simulink model "IEEE_39bus_genout"  (R2021a)
settings: Solver=ode3  StartTime=0.0  StopTime=100  FixedStep=Ts  MaxStep=1/60  RelTol=1e-2  AbsTol=1e-1
PreLoadFcn:
  | Ts=50e-6; ssn_ieee39_params; dec=20;
InitFcn:
  | Ts=50e-6; ssn_ieee39_params; dec=20;
values from neighbouring files (symbols this model uses):
  f = 50    [ssn_ieee39_params_ctrl.m]
  fNom = f    (= 60)    [ssn_ieee39_params_ctrl.m]
  ILR = 5.02    [ssn_ieee39_params_ctrl.m]
  IQMIN = 0.1    [ssn_ieee39_params_ctrl.m]
  ISCLIM = 1    [ssn_ieee39_params_ctrl.m]
  ITFpu = 1.10    (= 1.1)    [ssn_ieee39_params_ctrl.m]
  K = 1    [ssn_ieee39_params_ctrl.m]
  K1 = 1    [ssn_ieee39_params_ctrl.m]
  K2 = 2    [ssn_ieee39_params_ctrl.m]
  KCL = 1.04    [ssn_ieee39_params_ctrl.m]
  KFB = 0    [ssn_ieee39_params_ctrl.m]
  KFF = 1    [ssn_ieee39_params_ctrl.m]
  KFIX = 1    [ssn_ieee39_params_ctrl.m]
  KG = 1    [ssn_ieee39_params_ctrl.m]
  KIA = 59.91    [ssn_ieee39_params_ctrl.m]
  KIOEX = 0.0303    [ssn_ieee39_params_ctrl.m]
  KIUEX = 0.0303    [ssn_ieee39_params_ctrl.m]
  KIUOEX = 1    [ssn_ieee39_params_ctrl.m]
  KIUUEX = 1    [ssn_ieee39_params_ctrl.m]
  KLR = 22.47    [ssn_ieee39_params_ctrl.m]
  KM = 1    [ssn_ieee39_params_ctrl.m]
  KOEL = 0.24    [ssn_ieee39_params_ctrl.m]
  Kp = 1    [ssn_ieee39_params_ctrl.m]
  KPA = 30    [ssn_ieee39_params_ctrl.m]
  KPOEL = 1    [ssn_ieee39_params_ctrl.m]
  KPOEX = 0    [ssn_ieee39_params_ctrl.m]
  KPUEX = 0    [ssn_ieee39_params_ctrl.m]
  KSCALE = 0.319    [ssn_ieee39_params_ctrl.m]
  KUF = 0    [ssn_ieee39_params_ctrl.m]
  KUI = 0.001    [ssn_ieee39_params_ctrl.m]
  KUL = 0.24    [ssn_ieee39_params_ctrl.m]
  s = 10    [ssn_ieee39_params_ctrl.m]
  TA = 0.01    [ssn_ieee39_params_ctrl.m]
  Tadj = 0    [ssn_ieee39_params_ctrl.m]
  taps = [1 1 1.07 1.07 1.009 1.025 1 1.025 1.025 1.025]*1    [ssn_ieee39_params_ctrl.m]
  TF = 0.02    [ssn_ieee39_params_ctrl.m]
  TG = 0.024    [ssn_ieee39_params_ctrl.m]
  TINV = 0    [ssn_ieee39_params_ctrl.m]
  TIT = 0.1    [ssn_ieee39_params_ctrl.m]
  TL_10_11_len = 14    [ssn_ieee39_params_ctrl.m]
  TL_10_13_len = 14    [ssn_ieee39_params_ctrl.m]
  TL_13_14_len = 32    [ssn_ieee39_params_ctrl.m]
  TL_14_15_len = 70    [ssn_ieee39_params_ctrl.m]
  TL_15_16_len = 31.5    [ssn_ieee39_params_ctrl.m]
  TL_16_17_len = 26    [ssn_ieee39_params_ctrl.m]
  TL_16_19_len = 61    [ssn_ieee39_params_ctrl.m]
  TL_16_21_len = 46    [ssn_ieee39_params_ctrl.m]
  TL_16_24_len = 15    [ssn_ieee39_params_ctrl.m]
  TL_17_18_len = 26    [ssn_ieee39_params_ctrl.m]
  TL_17_27_len = 59    [ssn_ieee39_params_ctrl.m]
  TL_1_2_len = 134    [ssn_ieee39_params_ctrl.m]
  TL_1_39_len = 105    [ssn_ieee39_params_ctrl.m]
  TL_21_22_len = 47    [ssn_ieee39_params_ctrl.m]
  TL_22_23_len = 33    [ssn_ieee39_params_ctrl.m]
  TL_24_23_len = 88    [ssn_ieee39_params_ctrl.m]
  TL_25_26_len = 101    [ssn_ieee39_params_ctrl.m]
  TL_26_27_len = 46.5    [ssn_ieee39_params_ctrl.m]
  TL_26_28_len = 151    [ssn_ieee39_params_ctrl.m]
  TL_26_29_len = 200    [ssn_ieee39_params_ctrl.m]
  TL_28_29_len = 48    [ssn_ieee39_params_ctrl.m]
  TL_2_25_len = 28    [ssn_ieee39_params_ctrl.m]
  TL_2_2_len = 49    [ssn_ieee39_params_ctrl.m]
  TL_3_18_len = 42    [ssn_ieee39_params_ctrl.m]
  TL_3_4_len = 53    [ssn_ieee39_params_ctrl.m]
  TL_4_14_len = 33    [ssn_ieee39_params_ctrl.m]
  TL_4_5_len = 32.5    [ssn_ieee39_params_ctrl.m]
  TL_5_6_len = 14    [ssn_ieee39_params_ctrl.m]
  TL_5_8_len = 32    [ssn_ieee39_params_ctrl.m]
  TL_6_11_len = 26.5    [ssn_ieee39_params_ctrl.m]
  TL_6_7_len = 25.5    [ssn_ieee39_params_ctrl.m]
  TL_7_8_len = 15    [ssn_ieee39_params_ctrl.m]
  TL_8_9_len = 93    [ssn_ieee39_params_ctrl.m]
  TL_9_39_len = 136    [ssn_ieee39_params_ctrl.m]
  TOEL = 5.00    (= 5)    [ssn_ieee39_params_ctrl.m]
  TQREF = 0    [ssn_ieee39_params_ctrl.m]
  TQSCL = 0.012    [ssn_ieee39_params_ctrl.m]
  Ts_PMU = 1/1000    (= 0.001)    [ssn_ieee39_params_ctrl.m]
  TU1 = 0    [ssn_ieee39_params_ctrl.m]
  TU2 = 0    [ssn_ieee39_params_ctrl.m]
  TU3 = 0    [ssn_ieee39_params_ctrl.m]
  TU4 = 0    [ssn_ieee39_params_ctrl.m]
  TUL = 0    [ssn_ieee39_params_ctrl.m]
  TUP = 0.050    (= 0.05)    [ssn_ieee39_params_ctrl.m]
  TUQ = .005    (= 0.005)    [ssn_ieee39_params_ctrl.m]
  TUV = 0.2    [ssn_ieee39_params_ctrl.m]
  VAAMAX = VAMAX    (= 7.05)    [ssn_ieee39_params_ctrl.m]
  VAMAX = 7.05    [ssn_ieee39_params_ctrl.m]
  VAMIN = -6.11    [ssn_ieee39_params_ctrl.m]
  VBMAX = 999    [ssn_ieee39_params_ctrl.m]
  VF = 0    [ssn_ieee39_params_ctrl.m]
  VFB = 0    [ssn_ieee39_params_ctrl.m]
  VMMAX = 7.05    [ssn_ieee39_params_ctrl.m]
  VMMIN = -6.11    [ssn_ieee39_params_ctrl.m]
  VOELmax1 = 0.2353    [ssn_ieee39_params_ctrl.m]
  VOELmax2 = 0.0    (= 0)    [ssn_ieee39_params_ctrl.m]
  VOELmin1 = -0.24    [ssn_ieee39_params_ctrl.m]
  VOELmin2 = -1.0    (= -1)    [ssn_ieee39_params_ctrl.m]
  VRMAX = 7.05    [ssn_ieee39_params_ctrl.m]
  VRMIN = -6.11    [ssn_ieee39_params_ctrl.m]
  VSCLmax = 0.20    (= 0.2)    [ssn_ieee39_params_ctrl.m]
  VSCLmin = -0.10    (= -0.1)    [ssn_ieee39_params_ctrl.m]
  VUELmax1 = 1    [ssn_ieee39_params_ctrl.m]
  VUELmax2 = 1    [ssn_ieee39_params_ctrl.m]
  VUELmin1 = -1    [ssn_ieee39_params_ctrl.m]
  VUELmin2 = -1    [ssn_ieee39_params_ctrl.m]
  VUImax = 1    [ssn_ieee39_params_ctrl.m]
  VUImin = -1    [ssn_ieee39_params_ctrl.m]
undefined symbols (not defined in the file or in its folder): D1, Delta, MOV_segment9, powergui
libraries: spsThreePhaseVIMeasurementLib x42, slpidlib x40, powerlib_extras x30, op_dpl_lib x30, simulink_extras x20, spsST2AModel x20, spsThreePhaseParallelRLCLoadLib x19, spsThreePhaseTransformerTwoWindingsLib x13, spsSynchronousMachinepuStandardLib x10, simulink x10, spsPower3phInstantaneousLib x10, spsThreePhasePISectionLineLib x7
(part 4 of 12)

== system IEEE_39bus_genout/SM_master/PMU_Vpos_60Hz7 ==
  abc : Inport  PortDimensions=3
  1 / sqrt of 2 : Gain  Gain=1/sqrt(2)  OutDataTypeStr=Inherit: Same as input  ParamDataTypeStr=Inherit: Same as input
  Cartesian to Polar : simulink_extras/Transformations/Cartesian to Polar
  Demux : Demux  Outputs=3
      settings: DisplayOption=none
  Discrete Mean value1 : powerlib_extras/Discrete Measurements/Discrete  Mean value  Freq=Freq  Vinit=Real_Init  Ts=Ts
      settings: SourceProductBaseCode=PS
  Discrete Mean value2 : powerlib_extras/Discrete Measurements/Discrete  Mean value  Freq=Freq  Vinit=Imag_Init  Ts=Ts
      settings: SourceProductBaseCode=PS
  Discrete Derivative : simulink/Discrete/Discrete Derivative  gainval=1.0  ICPrevScaledInput=0.0  OutMin=[]  OutMax=[]  OutDataType=fixdt(1, 16)  OutScaling=2^-10  DoSatur=off
  Gain : Gain  Gain=2*pi*Freq  SaturateOnIntegerOverflow=on  OutDataTypeStr=Inherit: Same as input  ParamDataTypeStr=Inherit: Same as input
  Mux : Mux  Inputs=2
  Rad->Deg. : Gain  Gain=180/pi  SaturateOnIntegerOverflow=on  OutDataTypeStr=Inherit: Same as input  ParamDataTypeStr=Inherit: Same as input
  Sum : Sum  Inputs=|++  OutDataTypeStr=Inherit: Same as first input
  Terminator : Terminator
  Trigonometric Function : Trigonometry
  Trigonometric Function1 : Trigonometry  Operator=cos
  abc_to_dq0 Transformation : powerlib_extras/Measurements/abc_to_dq0 Transformation
      settings: SourceProductBaseCode=PS
  fo : Constant  Value=2*pi*Freq
  t : DigitalClock  SampleTime=Ts
  Mag : Outport
  Phase : Outport  Port=2
  freq : Outport  Port=3
  dfdt : Outport  Port=4
  wires:
  Cartesian to Polar/2 -> Rad->Deg./1, Discrete Derivative/1
  Gain/1 -> Trigonometric Function1/1, Trigonometric Function/1
  t/1 -> Gain/1
  abc/1 -> abc_to_dq0 Transformation/1
  Mux/1 -> abc_to_dq0 Transformation/2
  Discrete Mean value1/1 -> Cartesian to Polar/1  "Real"
  Rad->Deg./1 -> Phase/1
  Discrete Mean value2/1 -> Cartesian to Polar/2  "Real"
  abc_to_dq0 Transformation/1 -> Demux/1
  Demux/3 -> Terminator/1
  Demux/2 -> Discrete Mean value2/1
  Demux/1 -> Discrete Mean value1/1
  Trigonometric Function/1 -> Mux/1
  Trigonometric Function1/1 -> Mux/2
  Cartesian to Polar/1 -> 1 / sqrt of 2/1
  1 / sqrt of 2/1 -> Mag/1
  Discrete Derivative/1 -> Sum/2, dfdt/1
  fo/1 -> Sum/1
  Sum/1 -> freq/1

== system IEEE_39bus_genout/SM_master/PMU_Vpos_60Hz8 ==
  abc : Inport  PortDimensions=3
  1 / sqrt of 2 : Gain  Gain=1/sqrt(2)  OutDataTypeStr=Inherit: Same as input  ParamDataTypeStr=Inherit: Same as input
  Cartesian to Polar : simulink_extras/Transformations/Cartesian to Polar
  Demux : Demux  Outputs=3
      settings: DisplayOption=none
  Discrete Mean value1 : powerlib_extras/Discrete Measurements/Discrete  Mean value  Freq=Freq  Vinit=Real_Init  Ts=Ts
      settings: SourceProductBaseCode=PS
  Discrete Mean value2 : powerlib_extras/Discrete Measurements/Discrete  Mean value  Freq=Freq  Vinit=Imag_Init  Ts=Ts
      settings: SourceProductBaseCode=PS
  Discrete Derivative : simulink/Discrete/Discrete Derivative  gainval=1.0  ICPrevScaledInput=0.0  OutMin=[]  OutMax=[]  OutDataType=fixdt(1, 16)  OutScaling=2^-10  DoSatur=off
  Gain : Gain  Gain=2*pi*Freq  SaturateOnIntegerOverflow=on  OutDataTypeStr=Inherit: Same as input  ParamDataTypeStr=Inherit: Same as input
  Mux : Mux  Inputs=2
  Rad->Deg. : Gain  Gain=180/pi  SaturateOnIntegerOverflow=on  OutDataTypeStr=Inherit: Same as input  ParamDataTypeStr=Inherit: Same as input
  Sum : Sum  Inputs=|++  OutDataTypeStr=Inherit: Same as first input
  Terminator : Terminator
  Trigonometric Function : Trigonometry
  Trigonometric Function1 : Trigonometry  Operator=cos
  abc_to_dq0 Transformation : powerlib_extras/Measurements/abc_to_dq0 Transformation
      settings: SourceProductBaseCode=PS
  fo : Constant  Value=2*pi*Freq
  t : DigitalClock  SampleTime=Ts
  Mag : Outport
  Phase : Outport  Port=2
  freq : Outport  Port=3
  dfdt : Outport  Port=4
  wires:
  Cartesian to Polar/2 -> Rad->Deg./1, Discrete Derivative/1
  Gain/1 -> Trigonometric Function1/1, Trigonometric Function/1
  t/1 -> Gain/1
  abc/1 -> abc_to_dq0 Transformation/1
  Mux/1 -> abc_to_dq0 Transformation/2
  Discrete Mean value1/1 -> Cartesian to Polar/1  "Real"
  Rad->Deg./1 -> Phase/1
  Discrete Mean value2/1 -> Cartesian to Polar/2  "Real"
  abc_to_dq0 Transformation/1 -> Demux/1
  Demux/3 -> Terminator/1
  Demux/2 -> Discrete Mean value2/1
  Demux/1 -> Discrete Mean value1/1
  Trigonometric Function/1 -> Mux/1
  Trigonometric Function1/1 -> Mux/2
  Cartesian to Polar/1 -> 1 / sqrt of 2/1
  1 / sqrt of 2/1 -> Mag/1
  Discrete Derivative/1 -> Sum/2, dfdt/1
  fo/1 -> Sum/1
  Sum/1 -> freq/1

== system IEEE_39bus_genout/SM_master/PMU_Vpos_60Hz9 ==
  abc : Inport  PortDimensions=3
  1 / sqrt of 2 : Gain  Gain=1/sqrt(2)  OutDataTypeStr=Inherit: Same as input  ParamDataTypeStr=Inherit: Same as input
  Cartesian to Polar : simulink_extras/Transformations/Cartesian to Polar
  Demux : Demux  Outputs=3
      settings: DisplayOption=none
  Discrete Mean value1 : powerlib_extras/Discrete Measurements/Discrete  Mean value  Freq=Freq  Vinit=Real_Init  Ts=Ts
      settings: SourceProductBaseCode=PS
  Discrete Mean value2 : powerlib_extras/Discrete Measurements/Discrete  Mean value  Freq=Freq  Vinit=Imag_Init  Ts=Ts
      settings: SourceProductBaseCode=PS
  Discrete Derivative : simulink/Discrete/Discrete Derivative  gainval=1.0  ICPrevScaledInput=0.0  OutMin=[]  OutMax=[]  OutDataType=fixdt(1, 16)  OutScaling=2^-10  DoSatur=off
  Gain : Gain  Gain=2*pi*Freq  SaturateOnIntegerOverflow=on  OutDataTypeStr=Inherit: Same as input  ParamDataTypeStr=Inherit: Same as input
  Mux : Mux  Inputs=2
  Rad->Deg. : Gain  Gain=180/pi  SaturateOnIntegerOverflow=on  OutDataTypeStr=Inherit: Same as input  ParamDataTypeStr=Inherit: Same as input
  Sum : Sum  Inputs=|++  OutDataTypeStr=Inherit: Same as first input
  Terminator : Terminator
  Trigonometric Function : Trigonometry
  Trigonometric Function1 : Trigonometry  Operator=cos
  abc_to_dq0 Transformation : powerlib_extras/Measurements/abc_to_dq0 Transformation
      settings: SourceProductBaseCode=PS
  fo : Constant  Value=2*pi*Freq
  t : DigitalClock  SampleTime=Ts
  Mag : Outport
  Phase : Outport  Port=2
  freq : Outport  Port=3
  dfdt : Outport  Port=4
  wires:
  Cartesian to Polar/2 -> Rad->Deg./1, Discrete Derivative/1
  Gain/1 -> Trigonometric Function1/1, Trigonometric Function/1
  t/1 -> Gain/1
  abc/1 -> abc_to_dq0 Transformation/1
  Mux/1 -> abc_to_dq0 Transformation/2
  Discrete Mean value1/1 -> Cartesian to Polar/1  "Real"
  Rad->Deg./1 -> Phase/1
  Discrete Mean value2/1 -> Cartesian to Polar/2  "Real"
  abc_to_dq0 Transformation/1 -> Demux/1
  Demux/3 -> Terminator/1
  Demux/2 -> Discrete Mean value2/1
  Demux/1 -> Discrete Mean value1/1
  Trigonometric Function/1 -> Mux/1
  Trigonometric Function1/1 -> Mux/2
  Cartesian to Polar/1 -> 1 / sqrt of 2/1
  1 / sqrt of 2/1 -> Mag/1
  Discrete Derivative/1 -> Sum/2, dfdt/1
  fo/1 -> Sum/1
  Sum/1 -> freq/1

== system IEEE_39bus_genout/SM_master/Power ==
  Mux : Mux  Inputs=10
  Power (3ph, Instantaneous){1..10} (10 alike) : spsPower3phInstantaneousLib/Power (3ph, Instantaneous)
  Scope{1..10} (10 alike) : Scope  NumInputPorts=2
  to PU{1..20} (20 alike) : Gain
  Pgen : Outport
  tag scope: PG_10=global, PG_1=global, PG_2=global, PG_3=global, PG_4=global, PG_5=global, PG_6=global, PG_7=global, PG_8=global, PG_9=global
  wires:
  [Iabc_30] -> "Power (3ph, Instantaneous)1"/2
  to PU2/1 -> Scope7/2, [QG_10]
  [Vabc_30] -> "Power (3ph, Instantaneous)1"/1
  "Power (3ph, Instantaneous)4"/2 -> to PU9/1
  to PU8/1 -> [PG_8], Scope4/1
  "Power (3ph, Instantaneous)1"/1 -> to PU1/1
  "Power (3ph, Instantaneous)1"/2 -> to PU2/1
  "Power (3ph, Instantaneous)4"/1 -> to PU8/1
  [Vabc_37] -> "Power (3ph, Instantaneous)4"/1
  to PU1/1 -> Scope7/1, [PG_10]
  [Iabc_37] -> "Power (3ph, Instantaneous)4"/2
  to PU9/1 -> [QG_8], Scope4/2
  to PU6/1 -> Scope1/2, [QG_9]
  [Iabc_29] -> "Power (3ph, Instantaneous)3"/2
  to PU3/1 -> [PG_1], Scope2/1
  [Vabc_29] -> "Power (3ph, Instantaneous)3"/1
  "Power (3ph, Instantaneous)3"/1 -> to PU5/1
  "Power (3ph, Instantaneous)2"/2 -> to PU4/1
  "Power (3ph, Instantaneous)2"/1 -> to PU3/1
  to PU5/1 -> Scope1/1, [PG_9]
  "Power (3ph, Instantaneous)3"/2 -> to PU6/1
  [Vabc_391] -> "Power (3ph, Instantaneous)2"/1
  to PU4/1 -> [QG_1], Scope2/2
  [Iabc_391] -> "Power (3ph, Instantaneous)2"/2
  [Iabc_34] -> "Power (3ph, Instantaneous)6"/2
  to PU12/1 -> Scope5/2, [QG_5]
  [Vabc_34] -> "Power (3ph, Instantaneous)6"/1
  "Power (3ph, Instantaneous)7"/2 -> to PU14/1
  to PU13/1 -> [PG_4], Scope3/1
  "Power (3ph, Instantaneous)6"/1 -> to PU11/1
  "Power (3ph, Instantaneous)6"/2 -> to PU12/1
  "Power (3ph, Instantaneous)7"/1 -> to PU13/1
  [Vabc_33] -> "Power (3ph, Instantaneous)7"/1
  to PU11/1 -> Scope5/1, [PG_5]
  [Iabc_33] -> "Power (3ph, Instantaneous)7"/2
  to PU14/1 -> [QG_4], Scope3/2
  to PU16/1 -> Scope6/2, [QG_2]
  [Iabc_31] -> "Power (3ph, Instantaneous)8"/2
  to PU7/1 -> [PG_3], Scope8/1
  [Vabc_31] -> "Power (3ph, Instantaneous)8"/1
  "Power (3ph, Instantaneous)8"/1 -> to PU15/1
  "Power (3ph, Instantaneous)5"/2 -> to PU10/1
  "Power (3ph, Instantaneous)5"/1 -> to PU7/1
  to PU15/1 -> Scope6/1, [PG_2]
  "Power (3ph, Instantaneous)8"/2 -> to PU16/1
  [Vabc_32] -> "Power (3ph, Instantaneous)5"/1
  to PU10/1 -> [QG_3], Scope8/2
  [Iabc_32] -> "Power (3ph, Instantaneous)5"/2
  [Iabc_35] -> "Power (3ph, Instantaneous)9"/2
  to PU17/1 -> Scope10/2, [QG_6]
  [Vabc_35] -> "Power (3ph, Instantaneous)9"/1
  "Power (3ph, Instantaneous)9"/1 -> to PU20/1
  "Power (3ph, Instantaneous)9"/2 -> to PU17/1
  to PU20/1 -> Scope10/1, [PG_6]
  to PU18/1 -> [PG_7], Scope9/1
  "Power (3ph, Instantaneous)10"/2 -> to PU19/1
  "Power (3ph, Instantaneous)10"/1 -> to PU18/1
  [Vabc_36] -> "Power (3ph, Instantaneous)10"/1
  to PU19/1 -> [QG_7], Scope9/2
  [Iabc_36] -> "Power (3ph, Instantaneous)10"/2
  [PG_1] -> Mux/1
  [PG_2] -> Mux/2
  [PG_3] -> Mux/3
  [PG_4] -> Mux/4
  [PG_5] -> Mux/5
  [PG_6] -> Mux/6
  [PG_7] -> Mux/7
  [PG_8] -> Mux/8
  [PG_9] -> Mux/9
  [PG_10] -> Mux/10
  Mux/1 -> Pgen/1

== system IEEE_39bus_genout/SM_master/Snubber circuit ==
  Snubber 2 : spsThreePhaseSeriesRLCLoadLib/Three-Phase Series RLC Load  LConnTagsString=A|B|C  Configuration=Y (grounded)  NominalVoltage=20000  Vabc=[1e3 1e3 1e3]  Vabcp=[1e3 1e3 1e3]  NominalFrequency=60  UnbalancedPower=off  ActivePower=1e6  InductivePower=0  CapacitivePower=1e7  Pabc=[10e3 9e3 11e3]  QLabc=[100 90 110]  QCabc=[100 90 110]  Pabcp=[10e3 9e3 11e3]  QLabcp=[100 90 110]  QCabcp=[100 90 110]  Measurements=None  LoadType=constant Z
  Three-Phase Series RLC Branch : spsThreePhaseSeriesRLCBranchLib/Three-Phase Series RLC Branch  LConnTagsString=A|B|C  RConnTagsString=A|B|C  BranchType=R  Resistance=1e10  Inductance=1e-3  Capacitance=1e-6  Measurements=None
  a : PMIOPort  Side=Left
  b : PMIOPort  Port=2  Side=Left
  c : PMIOPort  Port=3  Side=Left
  Conn4 : PMIOPort  Port=4  Side=Right
  connections:
  Snubber 2/LConn3 -- c/RConn1 -- Three-Phase Series RLC Branch/LConn3
  Three-Phase Series RLC Branch/RConn2 -- Conn4/RConn1 -- Three-Phase Series RLC Branch/RConn3 -- Three-Phase Series RLC Branch/RConn1
  Three-Phase Series RLC Branch/LConn2 -- b/RConn1 -- Snubber 2/LConn2
  Three-Phase Series RLC Branch/LConn1 -- a/RConn1 -- Snubber 2/LConn1

== system IEEE_39bus_genout/powergui/EquivalentModel1 ==
  Sources : Subsystem
  State-Space : S-Function  FunctionName=ssn_sfun_v1  Parameters=1,0  SFunctionDeploymentMode=off  EnableBusSupport=off  SFcnStateName=MOV_segment9,MOV_segment9,MOV_segment9,MOV_segment9,MOV_segment9,MOV_segment9,MOV_segment9,MOV_segment9,MOV_segment9,MOV_segment9
      settings: SFcnIsStateOwnerBlock=on
  Yout : Subsystem
  wires:
  State-Space/1 -> Yout/1(v,i)
  Sources/1(u) -> State-Space/1

== system IEEE_39bus_genout/powergui/EquivalentModel10 ==
  Sources : Subsystem
  State-Space : S-Function  FunctionName=ssn_sfun_v1  Parameters=10,0  SFunctionDeploymentMode=off  EnableBusSupport=off  SFcnStateName=MOV_segment9,MOV_segment9,MOV_segment9,MOV_segment9,MOV_segment9,MOV_segment9,MOV_segment9,MOV_segment9,MOV_segment9,MOV_segment9
      settings: SFcnIsStateOwnerBlock=on
  Yout : Subsystem
  wires:
  State-Space/1 -> Yout/1(v,i)
  Sources/1(u) -> State-Space/1

== system IEEE_39bus_genout/powergui/EquivalentModel11 ==
  Sources : Subsystem
  State-Space : S-Function  FunctionName=ssn_sfun_v1  Parameters=11,0  SFunctionDeploymentMode=off  EnableBusSupport=off  SFcnStateName=MOV_segment9,MOV_segment9,MOV_segment9,MOV_segment9,MOV_segment9,MOV_segment9,MOV_segment9,MOV_segment9,MOV_segment9,MOV_segment9
      settings: SFcnIsStateOwnerBlock=on
  Yout : Subsystem
  wires:
  State-Space/1 -> Yout/1(v,i)
  Sources/1(u) -> State-Space/1

== system IEEE_39bus_genout/powergui/EquivalentModel12 ==
  Sources : Subsystem
  State-Space : S-Function  FunctionName=ssn_sfun_v1  Parameters=12,0  SFunctionDeploymentMode=off  EnableBusSupport=off  SFcnStateName=MOV_segment9,MOV_segment9,MOV_segment9,MOV_segment9,MOV_segment9,MOV_segment9,MOV_segment9,MOV_segment9,MOV_segment9,MOV_segment9
      settings: SFcnIsStateOwnerBlock=on
  Yout : Subsystem
  wires:
  State-Space/1 -> Yout/1(v,i)
  Sources/1(u) -> State-Space/1

== system IEEE_39bus_genout/powergui/EquivalentModel13 ==
  Sources : Subsystem
  State-Space : S-Function  FunctionName=ssn_sfun_v1  Parameters=13,0  SFunctionDeploymentMode=off  EnableBusSupport=off  SFcnStateName=MOV_segment9,MOV_segment9,MOV_segment9,MOV_segment9,MOV_segment9,MOV_segment9,MOV_segment9,MOV_segment9,MOV_segment9,MOV_segment9
      settings: SFcnIsStateOwnerBlock=on
  Yout : Subsystem
  wires:
  State-Space/1 -> Yout/1(v,i)
  Sources/1(u) -> State-Space/1

== system IEEE_39bus_genout/powergui/EquivalentModel14 ==
  Sources : Subsystem
  State-Space : S-Function  FunctionName=ssn_sfun_v1  Parameters=14,0  SFunctionDeploymentMode=off  EnableBusSupport=off  SFcnStateName=MOV_segment9,MOV_segment9,MOV_segment9,MOV_segment9,MOV_segment9,MOV_segment9,MOV_segment9,MOV_segment9,MOV_segment9,MOV_segment9
      settings: SFcnIsStateOwnerBlock=on
  Yout : Subsystem
  wires:
  State-Space/1 -> Yout/1(v,i)
  Sources/1(u) -> State-Space/1

== system IEEE_39bus_genout/powergui/EquivalentModel15 ==
  Sources : Subsystem
  State-Space : S-Function  FunctionName=ssn_sfun_v1  Parameters=15,0  SFunctionDeploymentMode=off  EnableBusSupport=off  SFcnStateName=MOV_segment9,MOV_segment9,MOV_segment9,MOV_segment9,MOV_segment9,MOV_segment9,MOV_segment9,MOV_segment9,MOV_segment9,MOV_segment9
      settings: SFcnIsStateOwnerBlock=on
  Yout : Subsystem
  wires:
  State-Space/1 -> Yout/1(v,i)
  Sources/1(u) -> State-Space/1

== system IEEE_39bus_genout/powergui/EquivalentModel16 ==
  Sources : Subsystem
  State-Space : S-Function  FunctionName=ssn_sfun_v1  Parameters=16,0  SFunctionDeploymentMode=off  EnableBusSupport=off  SFcnStateName=MOV_segment9,MOV_segment9,MOV_segment9,MOV_segment9,MOV_segment9,MOV_segment9,MOV_segment9,MOV_segment9,MOV_segment9,MOV_segment9
      settings: SFcnIsStateOwnerBlock=on
  Yout : Subsystem
  wires:
  State-Space/1 -> Yout/1(v,i)
  Sources/1(u) -> State-Space/1

== system IEEE_39bus_genout/powergui/EquivalentModel17 ==
  Sources : Subsystem
  State-Space : S-Function  FunctionName=ssn_sfun_v1  Parameters=17,0  SFunctionDeploymentMode=off  EnableBusSupport=off  SFcnStateName=MOV_segment9,MOV_segment9,MOV_segment9,MOV_segment9,MOV_segment9,MOV_segment9,MOV_segment9,MOV_segment9,MOV_segment9,MOV_segment9
      settings: SFcnIsStateOwnerBlock=on
  Yout : Subsystem
  wires:
  State-Space/1 -> Yout/1(v,i)
  Sources/1(u) -> State-Space/1

== system IEEE_39bus_genout/powergui/EquivalentModel18 ==
  Sources : Subsystem
  State-Space : S-Function  FunctionName=ssn_sfun_v1  Parameters=18,0  SFunctionDeploymentMode=off  EnableBusSupport=off  SFcnStateName=MOV_segment9,MOV_segment9,MOV_segment9,MOV_segment9,MOV_segment9,MOV_segment9,MOV_segment9,MOV_segment9,MOV_segment9,MOV_segment9
      settings: SFcnIsStateOwnerBlock=on
  Yout : Subsystem
  wires:
  State-Space/1 -> Yout/1(v,i)
  Sources/1(u) -> State-Space/1

== system IEEE_39bus_genout/powergui/EquivalentModel19 ==
  Gates : Subsystem
  Sources : Subsystem
  State-Space : S-Function  FunctionName=ssn_sfun_v1  Parameters=19,0  SFunctionDeploymentMode=off  EnableBusSupport=off  SFcnStateName=MOV_segment9,MOV_segment9,MOV_segment9,MOV_segment9,MOV_segment9,MOV_segment9,MOV_segment9,MOV_segment9,MOV_segment9,MOV_segment9
      settings: SFcnIsStateOwnerBlock=on
  Status : Subsystem
  Yout : Subsystem
  wires:
  Gates/1(gates) -> State-Space/2
  Sources/1(u) -> State-Space/1
  State-Space/2 -> Status/1(status)
  State-Space/1 -> Yout/1(v,i)

== system IEEE_39bus_genout/powergui/EquivalentModel2 ==
  Sources : Subsystem
  State-Space : S-Function  FunctionName=ssn_sfun_v1  Parameters=2,0  SFunctionDeploymentMode=off  EnableBusSupport=off  SFcnStateName=MOV_segment9,MOV_segment9,MOV_segment9,MOV_segment9,MOV_segment9,MOV_segment9,MOV_segment9,MOV_segment9,MOV_segment9,MOV_segment9
      settings: SFcnIsStateOwnerBlock=on
  Yout : Subsystem
  wires:
  State-Space/1 -> Yout/1(v,i)
  Sources/1(u) -> State-Space/1

== system IEEE_39bus_genout/powergui/EquivalentModel20 ==
  Sources : Subsystem
  State-Space : S-Function  FunctionName=ssn_sfun_v1  Parameters=20,0  SFunctionDeploymentMode=off  EnableBusSupport=off  SFcnStateName=MOV_segment9,MOV_segment9,MOV_segment9,MOV_segment9,MOV_segment9,MOV_segment9,MOV_segment9,MOV_segment9,MOV_segment9,MOV_segment9
      settings: SFcnIsStateOwnerBlock=on
  Yout : Subsystem
  wires:
  State-Space/1 -> Yout/1(v,i)
  Sources/1(u) -> State-Space/1

== system IEEE_39bus_genout/powergui/EquivalentModel21 ==
  Sources : Subsystem
  State-Space : S-Function  FunctionName=ssn_sfun_v1  Parameters=21,0  SFunctionDeploymentMode=off  EnableBusSupport=off  SFcnStateName=MOV_segment9,MOV_segment9,MOV_segment9,MOV_segment9,MOV_segment9,MOV_segment9,MOV_segment9,MOV_segment9,MOV_segment9,MOV_segment9
      settings: SFcnIsStateOwnerBlock=on
  Yout : Subsystem
  wires:
  State-Space/1 -> Yout/1(v,i)
  Sources/1(u) -> State-Space/1

== system IEEE_39bus_genout/powergui/EquivalentModel22 ==
  Sources : Subsystem
  State-Space : S-Function  FunctionName=ssn_sfun_v1  Parameters=22,0  SFunctionDeploymentMode=off  EnableBusSupport=off  SFcnStateName=MOV_segment9,MOV_segment9,MOV_segment9,MOV_segment9,MOV_segment9,MOV_segment9,MOV_segment9,MOV_segment9,MOV_segment9,MOV_segment9
      settings: SFcnIsStateOwnerBlock=on
  Yout : Subsystem
  wires:
  State-Space/1 -> Yout/1(v,i)
  Sources/1(u) -> State-Space/1

== system IEEE_39bus_genout/powergui/EquivalentModel23 ==
  Sources : Subsystem
  State-Space : S-Function  FunctionName=ssn_sfun_v1  Parameters=23,0  SFunctionDeploymentMode=off  EnableBusSupport=off  SFcnStateName=MOV_segment9,MOV_segment9,MOV_segment9,MOV_segment9,MOV_segment9,MOV_segment9,MOV_segment9,MOV_segment9,MOV_segment9,MOV_segment9
      settings: SFcnIsStateOwnerBlock=on
  Yout : Subsystem
  wires:
  State-Space/1 -> Yout/1(v,i)
  Sources/1(u) -> State-Space/1

== system IEEE_39bus_genout/powergui/EquivalentModel24 ==
  Sources : Subsystem
  State-Space : S-Function  FunctionName=ssn_sfun_v1  Parameters=24,0  SFunctionDeploymentMode=off  EnableBusSupport=off  SFcnStateName=MOV_segment9,MOV_segment9,MOV_segment9,MOV_segment9,MOV_segment9,MOV_segment9,MOV_segment9,MOV_segment9,MOV_segment9,MOV_segment9
      settings: SFcnIsStateOwnerBlock=on
  Yout : Subsystem
  wires:
  State-Space/1 -> Yout/1(v,i)
  Sources/1(u) -> State-Space/1

== system IEEE_39bus_genout/powergui/EquivalentModel3 ==
  Sources : Subsystem
  State-Space : S-Function  FunctionName=ssn_sfun_v1  Parameters=3,0  SFunctionDeploymentMode=off  EnableBusSupport=off  SFcnStateName=MOV_segment9,MOV_segment9,MOV_segment9,MOV_segment9,MOV_segment9,MOV_segment9,MOV_segment9,MOV_segment9,MOV_segment9,MOV_segment9
      settings: SFcnIsStateOwnerBlock=on
  Yout : Subsystem
  wires:
  State-Space/1 -> Yout/1(v,i)
  Sources/1(u) -> State-Space/1

== system IEEE_39bus_genout/powergui/EquivalentModel4 ==
  Sources : Subsystem
  State-Space : S-Function  FunctionName=ssn_sfun_v1  Parameters=4,0  SFunctionDeploymentMode=off  EnableBusSupport=off  SFcnStateName=MOV_segment9,MOV_segment9,MOV_segment9,MOV_segment9,MOV_segment9,MOV_segment9,MOV_segment9,MOV_segment9,MOV_segment9,MOV_segment9
      settings: SFcnIsStateOwnerBlock=on
  Yout : Subsystem
  wires:
  State-Space/1 -> Yout/1(v,i)
  Sources/1(u) -> State-Space/1

== system IEEE_39bus_genout/powergui/EquivalentModel5 ==
  Sources : Subsystem
  State-Space : S-Function  FunctionName=ssn_sfun_v1  Parameters=5,0  SFunctionDeploymentMode=off  EnableBusSupport=off  SFcnStateName=MOV_segment9,MOV_segment9,MOV_segment9,MOV_segment9,MOV_segment9,MOV_segment9,MOV_segment9,MOV_segment9,MOV_segment9,MOV_segment9
      settings: SFcnIsStateOwnerBlock=on
  Yout : Subsystem
  wires:
  State-Space/1 -> Yout/1(v,i)
  Sources/1(u) -> State-Space/1

== system IEEE_39bus_genout/powergui/EquivalentModel6 ==
  Sources : Subsystem
  State-Space : S-Function  FunctionName=ssn_sfun_v1  Parameters=6,0  SFunctionDeploymentMode=off  EnableBusSupport=off  SFcnStateName=MOV_segment9,MOV_segment9,MOV_segment9,MOV_segment9,MOV_segment9,MOV_segment9,MOV_segment9,MOV_segment9,MOV_segment9,MOV_segment9
      settings: SFcnIsStateOwnerBlock=on
  Yout : Subsystem
  wires:
  State-Space/1 -> Yout/1(v,i)
  Sources/1(u) -> State-Space/1

== system IEEE_39bus_genout/powergui/EquivalentModel7 ==
  Sources : Subsystem
  State-Space : S-Function  FunctionName=ssn_sfun_v1  Parameters=7,0  SFunctionDeploymentMode=off  EnableBusSupport=off  SFcnStateName=MOV_segment9,MOV_segment9,MOV_segment9,MOV_segment9,MOV_segment9,MOV_segment9,MOV_segment9,MOV_segment9,MOV_segment9,MOV_segment9
      settings: SFcnIsStateOwnerBlock=on
  Yout : Subsystem
  wires:
  State-Space/1 -> Yout/1(v,i)
  Sources/1(u) -> State-Space/1

== system IEEE_39bus_genout/powergui/EquivalentModel8 ==
  Sources : Subsystem
  State-Space : S-Function  FunctionName=ssn_sfun_v1  Parameters=8,0  SFunctionDeploymentMode=off  EnableBusSupport=off  SFcnStateName=MOV_segment9,MOV_segment9,MOV_segment9,MOV_segment9,MOV_segment9,MOV_segment9,MOV_segment9,MOV_segment9,MOV_segment9,MOV_segment9
      settings: SFcnIsStateOwnerBlock=on
  Yout : Subsystem
  wires:
  State-Space/1 -> Yout/1(v,i)
  Sources/1(u) -> State-Space/1

== system IEEE_39bus_genout/powergui/EquivalentModel9 ==
  Sources : Subsystem
  State-Space : S-Function  FunctionName=ssn_sfun_v1  Parameters=9,0  SFunctionDeploymentMode=off  EnableBusSupport=off  SFcnStateName=MOV_segment9,MOV_segment9,MOV_segment9,MOV_segment9,MOV_segment9,MOV_segment9,MOV_segment9,MOV_segment9,MOV_segment9,MOV_segment9
      settings: SFcnIsStateOwnerBlock=on
  Yout : Subsystem
  wires:
  State-Space/1 -> Yout/1(v,i)
  Sources/1(u) -> State-Space/1

== system IEEE_39bus_genout/SM_master/G1/G1 ==
  note: Reactive Power
  note: Field Current
  note: Stator Current
  note: Stator Voltage
  note: Active Power
  note: Rotor Speed
  note: Measurement Outputs
  note: Mechanical
      | Power (Pm)
  note: Field Voltage (Vf)
  note: Stator Current
  note: Reactive Power
  note: Stator Voltage
  note: Voltage Reference
  note: Field Current
  note: Active Power
  note: SM Measurement Signal
  note: Rotor Speed Reference
  note: Rotor Speed
  wref (pu) : Inport
  Vref (pu) : Inport  Port=2
  Generator Measurements (Output) : Subsystem
  Governor model with Droop : Subsystem
  Ground7 : Ground
  ST6C EXCITER-1 : Subsystem
  Synchronous Machine : spsSynchronousMachinepuStandardLib/Synchronous Machine pu Standard  PresetModel=No  MechanicalLoad=Mechanical power Pm  ShowDetailedParameters=on  RotorType=Salient-pole  Units=per unit standard parameters  MeasurementBus=off  NominalParameters="[ Pn  Vn   f ]"  Reactances1=[ 31 32 33 34 35 36 37 ]  Reactances2=[ 1.305, 0.296, 0.252, 0.474, 0.243, 0.18 ]  dAxisTimeConstants=Short-circuit  qAxisTimeConstants=Open-circuit  TimeConstants1=[]  TimeConstants2=[]  TimeConstants3=[]  TimeConstants4=[]  TimeConstants5=[ 1.01, 0.053, 0.1 ]  TimeConstants6=[]  TimeConstants7=[]  TimeConstants8=[]  StatorResistance=2.8544e-3  Mechanical=[H1 0 2]  PolePairs=2  InitialConditions=[0 -62.5202 1.01055 1.01055 1.01055 8.25986 -111.74 128.26 1.32748]  SetSaturation=off  Saturation=[0.6404,0.7127,0.8441,0.9214,0.9956,1.082,1.19,1.316,1.457;0.7,0.7698,0.8872,0.9466,0.9969,1.046,1.1,1.151,1.201]  LoadFlowParameters=[1 150000000 0 0]  TsPowergui=0  TsBlock=-1  IterativeModel=Trapezoidal non iterative  IterativeDiscreteModel=Trapezoidal non iterative  BusType=PV  Pref=42e6  Qref=0  Qmin=-50000000  Qmax=50000000  PLF=0  QLF=0
      settings: SourceProductBaseCode=PS
  A : PMIOPort  Side=Right
  B : PMIOPort  Port=2  Side=Right
  C : PMIOPort  Port=3  Side=Right
  sm1 : Outport  VectorParamsAs1DForOutWhenUnconnected=off
  wires:
  Synchronous Machine/1 -> Generator Measurements (Output)/1(m)
  Vref (pu)/1 -> ST6C EXCITER-1/1(Vref)
  Governor model with Droop/1(Pmec (pu)) -> Synchronous Machine/1
  wref (pu)/1 -> Governor model with Droop/1(wref (pu)1)
  Ground7/1 -> ST6C EXCITER-1/5(Vstab)
  [QT1st] -> ST6C EXCITER-1/6(QT)
  [It1st] -> ST6C EXCITER-1/3(It)
  [PT1st] -> ST6C EXCITER-1/7(PT)
  ST6C EXCITER-1/1(Efd) -> [Efd1st], Synchronous Machine/2
  Generator Measurements (Output)/2(wm) -> [wm1]
  Generator Measurements (Output)/4(Ifd) -> [Ifd1st]
  Generator Measurements (Output)/5(It) -> [It1st]
  Generator Measurements (Output)/1(sm) -> sm1/1
  Generator Measurements (Output)/7(QT) -> [QT1st]
  Generator Measurements (Output)/6(PT) -> [PT1st]
  Generator Measurements (Output)/3(Vt) -> [Vt1st]
  [wm1] -> Governor model with Droop/2(w (pu))
  [Vt1st] -> ST6C EXCITER-1/2(Vt)
  [Ifd1st] -> ST6C EXCITER-1/4(Ifd)
  [PT1st] -> Governor model with Droop/3(Input)
  connections:
  B/RConn1 -- Synchronous Machine/RConn2
  C/RConn1 -- Synchronous Machine/RConn3
  A/RConn1 -- Synchronous Machine/RConn1

== system IEEE_39bus_genout/SM_master/G10/G10 ==
  note: Rotor Speed
  note: Rotor Speed Reference
  note: SM Measurement Signal
  note: Active Power
  note: Field Current
  note: Voltage Reference
  note: Stator Voltage
  note: Reactive Power
  note: Stator Current
  note: Field Voltage (Vf)
  note: Mechanical
      | Power (Pm)
  note: Measurement Outputs
  note: Rotor Speed
  note: Active Power
  note: Stator Voltage
  note: Stator Current
  note: Field Current
  note: Reactive Power
  wref (pu) : Inport
  Vref (pu) : Inport  Port=2
  "Generator Measurements " : Subsystem
  "Governor model " : Subsystem
  Ground7 : Ground
  ST6C EXCITER-1 : Subsystem
  Synchronous Machine : spsSynchronousMachinepuStandardLib/Synchronous Machine pu Standard  PresetModel=No  MechanicalLoad=Mechanical power Pm  ShowDetailedParameters=on  RotorType=Salient-pole  Units=per unit standard parameters  MeasurementBus=off  NominalParameters="[ Pn  Vn   f ]"  Reactances1=[ 31 32 33 34 35 36 37 ]  Reactances2=[ 1.305, 0.296, 0.252, 0.474, 0.243, 0.18 ]  dAxisTimeConstants=Short-circuit  qAxisTimeConstants=Open-circuit  TimeConstants1=[]  TimeConstants2=[]  TimeConstants3=[]  TimeConstants4=[]  TimeConstants5=[ 1.01, 0.053, 0.1 ]  TimeConstants6=[]  TimeConstants7=[]  TimeConstants8=[]  StatorResistance=2.8544e-3  Mechanical=[H1 0 2]  PolePairs=2  InitialConditions=[0 -62.5202 1.01055 1.01055 1.01055 8.25986 -111.74 128.26 1.32748]  SetSaturation=off  Saturation=[0.6404,0.7127,0.8441,0.9214,0.9956,1.082,1.19,1.316,1.457;0.7,0.7698,0.8872,0.9466,0.9969,1.046,1.1,1.151,1.201]  LoadFlowParameters=[1 150000000 0 0]  TsPowergui=0  TsBlock=-1  IterativeModel=Trapezoidal non iterative  IterativeDiscreteModel=Trapezoidal non iterative  BusType=PV  Pref=42e6  Qref=0  Qmin=-50000000  Qmax=50000000  PLF=0  QLF=0
      settings: SourceProductBaseCode=PS
  A : PMIOPort  Side=Right
  B : PMIOPort  Port=2  Side=Right
  C : PMIOPort  Port=3  Side=Right
  sm1 : Outport  VectorParamsAs1DForOutWhenUnconnected=off
  wires:
  [PT1st] -> "Governor model "/3(Input)
  [Ifd1st] -> ST6C EXCITER-1/4(Ifd)
  [Vt1st] -> ST6C EXCITER-1/2(Vt)
  [wm1] -> "Governor model "/2(w (pu))
  "Generator Measurements "/3(Vt) -> [Vt1st]
  "Generator Measurements "/6(PT) -> [PT1st]
  "Generator Measurements "/7(QT) -> [QT1st]
  "Generator Measurements "/1(sm) -> sm1/1
  "Generator Measurements "/5(It) -> [It1st]
  "Generator Measurements "/4(Ifd) -> [Ifd1st]
  "Generator Measurements "/2(wm) -> [wm1]
  ST6C EXCITER-1/1(Efd) -> Synchronous Machine/2, [Efd1st]
  [PT1st] -> ST6C EXCITER-1/7(PT)
  [It1st] -> ST6C EXCITER-1/3(It)
  [QT1st] -> ST6C EXCITER-1/6(QT)
  Ground7/1 -> ST6C EXCITER-1/5(Vstab)
  wref (pu)/1 -> "Governor model "/1(wref (pu)1)
  "Governor model "/1(Pmec (pu)) -> Synchronous Machine/1
  Vref (pu)/1 -> ST6C EXCITER-1/1(Vref)
  Synchronous Machine/1 -> "Generator Measurements "/1(m)
  connections:
  A/RConn1 -- Synchronous Machine/RConn1
  C/RConn1 -- Synchronous Machine/RConn3
  B/RConn1 -- Synchronous Machine/RConn2

== system IEEE_39bus_genout/SM_master/G2/G2 ==
  note: Reactive Power
  note: Field Current
  note: Stator Current
  note: Stator Voltage
  note: Active Power
  note: Rotor Speed
  note: Measurement Outputs
  note: Mechanical
      | Power (Pm)
  note: Field Voltage (Vf)
  note: Stator Current
  note: Reactive Power
  note: Stator Voltage
  note: Voltage Reference
  note: Field Current
  note: Active Power
  note: SM Measurement Signal
  note: Rotor Speed Reference
  note: Rotor Speed
  wref (pu) : Inport
  Vref (pu) : Inport  Port=2
  Generator Measurements (Output) : Subsystem
  "Governor model " : Subsystem
  Ground7 : Ground
  ST6C EXCITER-1 : Subsystem
  Synchronous Machine : spsSynchronousMachinepuStandardLib/Synchronous Machine pu Standard  PresetModel=No  MechanicalLoad=Mechanical power Pm  ShowDetailedParameters=on  RotorType=Salient-pole  Units=per unit standard parameters  MeasurementBus=off  NominalParameters="[ Pn  Vn   f ]"  Reactances1=[ 31 32 33 34 35 36 37 ]  Reactances2=[ 1.305, 0.296, 0.252, 0.474, 0.243, 0.18 ]  dAxisTimeConstants=Short-circuit  qAxisTimeConstants=Open-circuit  TimeConstants1=[]  TimeConstants2=[]  TimeConstants3=[]  TimeConstants4=[]  TimeConstants5=[ 1.01, 0.053, 0.1 ]  TimeConstants6=[]  TimeConstants7=[]  TimeConstants8=[]  StatorResistance=2.8544e-3  Mechanical=[H1 0 2]  PolePairs=2  InitialConditions=[0 -62.5202 1.01055 1.01055 1.01055 8.25986 -111.74 128.26 1.32748]  SetSaturation=off  Saturation=[0.6404,0.7127,0.8441,0.9214,0.9956,1.082,1.19,1.316,1.457;0.7,0.7698,0.8872,0.9466,0.9969,1.046,1.1,1.151,1.201]  LoadFlowParameters=[1 150000000 0 0]  TsPowergui=0  TsBlock=-1  IterativeModel=Trapezoidal non iterative  IterativeDiscreteModel=Trapezoidal non iterative  BusType=PV  Pref=42e6  Qref=0  Qmin=-50000000  Qmax=50000000  PLF=0  QLF=0
      settings: SourceProductBaseCode=PS
  A : PMIOPort  Side=Right
  B : PMIOPort  Port=2  Side=Right
  C : PMIOPort  Port=3  Side=Right
  sm1 : Outport  VectorParamsAs1DForOutWhenUnconnected=off
  wires:
  Synchronous Machine/1 -> Generator Measurements (Output)/1(m)
  Vref (pu)/1 -> ST6C EXCITER-1/1(Vref)
  "Governor model "/1(Pmec (pu)) -> Synchronous Machine/1
  wref (pu)/1 -> "Governor model "/1(wref (pu)1)
  Ground7/1 -> ST6C EXCITER-1/5(Vstab)
  [QT1st] -> ST6C EXCITER-1/6(QT)
  [It1st] -> ST6C EXCITER-1/3(It)
  [PT1st] -> ST6C EXCITER-1/7(PT)
  ST6C EXCITER-1/1(Efd) -> [Efd1st], Synchronous Machine/2
  Generator Measurements (Output)/2(wm) -> [wm1]
  Generator Measurements (Output)/4(Ifd) -> [Ifd1st]
  Generator Measurements (Output)/5(It) -> [It1st]
  Generator Measurements (Output)/1(sm) -> sm1/1
  Generator Measurements (Output)/7(QT) -> [QT1st]
  Generator Measurements (Output)/6(PT) -> [PT1st]
  Generator Measurements (Output)/3(Vt) -> [Vt1st]
  [wm1] -> "Governor model "/2(w (pu))
  [Vt1st] -> ST6C EXCITER-1/2(Vt)
  [Ifd1st] -> ST6C EXCITER-1/4(Ifd)
  [PT1st] -> "Governor model "/3(Input)
  connections:
  B/RConn1 -- Synchronous Machine/RConn2
  C/RConn1 -- Synchronous Machine/RConn3
  A/RConn1 -- Synchronous Machine/RConn1

== system IEEE_39bus_genout/SM_master/G3/G3 ==
  note: Rotor Speed
  note: Rotor Speed Reference
  note: SM Measurement Signal
  note: Active Power
  note: Field Current
  note: Voltage Reference
  note: Stator Voltage
  note: Reactive Power
  note: Stator Current
  note: Field Voltage (Vf)
  note: Synchronous
      | Machine
      | - Phase A
      | - Phase B
      | - Phase C
  note: Mechanical
      | Power (Pm)
  note: Selected (Combined)
      | Synchronous Machine
      | Measurement Outputs
  note: Rotor Speed
  note: Active Power
  note: Stator Voltage
  note: Stator Current
  note: Field Current
  note: Reactive Power
  wref (pu) : Inport
  Vref (pu) : Inport  Port=2
  Generator Measurements (Output) : Subsystem
  Governor model with Droop : Subsystem
  Ground7 : Ground
  ST6C EXCITER-1 : Subsystem
  Synchronous Machine : spsSynchronousMachinepuStandardLib/Synchronous Machine pu Standard  PresetModel=No  MechanicalLoad=Mechanical power Pm  ShowDetailedParameters=on  RotorType=Salient-pole  Units=per unit standard parameters  MeasurementBus=off  NominalParameters="[ Pn  Vn   f ]"  Reactances1=[ 31 32 33 34 35 36 37 ]  Reactances2=[ 1.305, 0.296, 0.252, 0.474, 0.243, 0.18 ]  dAxisTimeConstants=Short-circuit  qAxisTimeConstants=Open-circuit  TimeConstants1=[]  TimeConstants2=[]  TimeConstants3=[]  TimeConstants4=[]  TimeConstants5=[ 1.01, 0.053, 0.1 ]  TimeConstants6=[]  TimeConstants7=[]  TimeConstants8=[]  StatorResistance=2.8544e-3  Mechanical=[H1 0 2]  PolePairs=2  InitialConditions=[0 -62.5202 1.01055 1.01055 1.01055 8.25986 -111.74 128.26 1.32748]  SetSaturation=off  Saturation=[0.6404,0.7127,0.8441,0.9214,0.9956,1.082,1.19,1.316,1.457;0.7,0.7698,0.8872,0.9466,0.9969,1.046,1.1,1.151,1.201]  LoadFlowParameters=[1 150000000 0 0]  TsPowergui=0  TsBlock=-1  IterativeModel=Trapezoidal non iterative  IterativeDiscreteModel=Trapezoidal non iterative  BusType=PV  Pref=42e6  Qref=0  Qmin=-50000000  Qmax=50000000  PLF=0  QLF=0
      settings: SourceProductBaseCode=PS
  A : PMIOPort  Side=Right
  B : PMIOPort  Port=2  Side=Right
  C : PMIOPort  Port=3  Side=Right
  sm1 : Outport  VectorParamsAs1DForOutWhenUnconnected=off
  wires:
  [PT1st] -> Governor model with Droop/3(Input)
  [Ifd1st] -> ST6C EXCITER-1/4(Ifd)
  [Vt1st] -> ST6C EXCITER-1/2(Vt)
  [wm1] -> Governor model with Droop/2(w (pu))
  Generator Measurements (Output)/3(Vt) -> [Vt1st]
  Generator Measurements (Output)/6(PT) -> [PT1st]
  Generator Measurements (Output)/7(QT) -> [QT1st]
  Generator Measurements (Output)/1(sm) -> sm1/1
  Generator Measurements (Output)/5(It) -> [It1st]
  Generator Measurements (Output)/4(Ifd) -> [Ifd1st]
  Generator Measurements (Output)/2(wm) -> [wm1]
  ST6C EXCITER-1/1(Efd) -> Synchronous Machine/2, [Efd1st]
  [PT1st] -> ST6C EXCITER-1/7(PT)
  [It1st] -> ST6C EXCITER-1/3(It)
  [QT1st] -> ST6C EXCITER-1/6(QT)
  Ground7/1 -> ST6C EXCITER-1/5(Vstab)
  wref (pu)/1 -> Governor model with Droop/1(wref (pu)1)
  Governor model with Droop/1(Pmec (pu)) -> Synchronous Machine/1
  Vref (pu)/1 -> ST6C EXCITER-1/1(Vref)
  Synchronous Machine/1 -> Generator Measurements (Output)/1(m)
  connections:
  A/RConn1 -- Synchronous Machine/RConn1
  C/RConn1 -- Synchronous Machine/RConn3
  B/RConn1 -- Synchronous Machine/RConn2

== system IEEE_39bus_genout/SM_master/G4/G4 ==
  note: Rotor Speed
  note: Rotor Speed Reference
  note: SM Measurement Signal
  note: Active Power
  note: Field Current
  note: Voltage Reference
  note: Stator Voltage
  note: Reactive Power
  note: Stator Current
  note: Field Voltage (Vf)
  note: Mechanical
      | Power (Pm)
  note: Measurement Outputs
  note: Rotor Speed
  note: Active Power
  note: Stator Voltage
  note: Stator Current
  note: Field Current
  note: Reactive Power
  wref (pu) : Inport
  Vref (pu) : Inport  Port=2
  Generator Measurements (Output) : Subsystem
  "Governor model " : Subsystem
  Ground7 : Ground
  ST6C EXCITER-1 : Subsystem
  Synchronous Machine : spsSynchronousMachinepuStandardLib/Synchronous Machine pu Standard  PresetModel=No  MechanicalLoad=Mechanical power Pm  ShowDetailedParameters=on  RotorType=Salient-pole  Units=per unit standard parameters  MeasurementBus=off  NominalParameters="[ Pn  Vn   f ]"  Reactances1=[ 31 32 33 34 35 36 37 ]  Reactances2=[ 1.305, 0.296, 0.252, 0.474, 0.243, 0.18 ]  dAxisTimeConstants=Short-circuit  qAxisTimeConstants=Open-circuit  TimeConstants1=[]  TimeConstants2=[]  TimeConstants3=[]  TimeConstants4=[]  TimeConstants5=[ 1.01, 0.053, 0.1 ]  TimeConstants6=[]  TimeConstants7=[]  TimeConstants8=[]  StatorResistance=2.8544e-3  Mechanical=[H1 0 2]  PolePairs=2  InitialConditions=[0 -62.5202 1.01055 1.01055 1.01055 8.25986 -111.74 128.26 1.32748]  SetSaturation=off  Saturation=[0.6404,0.7127,0.8441,0.9214,0.9956,1.082,1.19,1.316,1.457;0.7,0.7698,0.8872,0.9466,0.9969,1.046,1.1,1.151,1.201]  LoadFlowParameters=[1 150000000 0 0]  TsPowergui=0  TsBlock=-1  IterativeModel=Trapezoidal non iterative  IterativeDiscreteModel=Trapezoidal non iterative  BusType=PV  Pref=42e6  Qref=0  Qmin=-50000000  Qmax=50000000  PLF=0  QLF=0
      settings: SourceProductBaseCode=PS
  A : PMIOPort  Side=Right
  B : PMIOPort  Port=2  Side=Right
  C : PMIOPort  Port=3  Side=Right
  sm1 : Outport  VectorParamsAs1DForOutWhenUnconnected=off
  wires:
  [PT1st] -> "Governor model "/3(Input)
  [Ifd1st] -> ST6C EXCITER-1/4(Ifd)
  [Vt1st] -> ST6C EXCITER-1/2(Vt)
  [wm1] -> "Governor model "/2(w (pu))
  Generator Measurements (Output)/3(Vt) -> [Vt1st]
  Generator Measurements (Output)/6(PT) -> [PT1st]
  Generator Measurements (Output)/7(QT) -> [QT1st]
  Generator Measurements (Output)/1(sm) -> sm1/1
  Generator Measurements (Output)/5(It) -> [It1st]
  Generator Measurements (Output)/4(Ifd) -> [Ifd1st]
  Generator Measurements (Output)/2(wm) -> [wm1]
  ST6C EXCITER-1/1(Efd) -> Synchronous Machine/2, [Efd1st]
  [PT1st] -> ST6C EXCITER-1/7(PT)
  [It1st] -> ST6C EXCITER-1/3(It)
  [QT1st] -> ST6C EXCITER-1/6(QT)
  Ground7/1 -> ST6C EXCITER-1/5(Vstab)
  wref (pu)/1 -> "Governor model "/1(wref (pu)1)
  "Governor model "/1(Pmec (pu)) -> Synchronous Machine/1
  Vref (pu)/1 -> ST6C EXCITER-1/1(Vref)
  Synchronous Machine/1 -> Generator Measurements (Output)/1(m)
  connections:
  A/RConn1 -- Synchronous Machine/RConn1
  C/RConn1 -- Synchronous Machine/RConn3
  B/RConn1 -- Synchronous Machine/RConn2

== system IEEE_39bus_genout/SM_master/G5/G5 ==
  note: Reactive Power
  note: Field Current
  note: Stator Current
  note: Stator Voltage
  note: Active Power
  note: Rotor Speed
  note: Selected (Combined)
      | Synchronous Machine
      | Measurement Outputs
  note: Mechanical
      | Power (Pm)
  note: Synchronous
      | Machine
      | - Phase A
      | - Phase B
      | - Phase C
  note: Field Voltage (Vf)
  note: Stator Current
  note: Reactive Power
  note: Stator Voltage
  note: Voltage Reference
  note: Field Current
  note: Active Power
  note: SM Measurement Signal
  note: Rotor Speed Reference
  note: Rotor Speed
  wref (pu) : Inport
  Vref (pu) : Inport  Port=2
  Generator Measurements (Output) : Subsystem
  Governor model with Droop : Subsystem
  Ground7 : Ground
  ST6C EXCITER-1 : Subsystem
  Synchronous Machine : spsSynchronousMachinepuStandardLib/Synchronous Machine pu Standard  PresetModel=No  MechanicalLoad=Mechanical power Pm  ShowDetailedParameters=on  RotorType=Salient-pole  Units=per unit standard parameters  MeasurementBus=off  NominalParameters="[ Pn  Vn   f ]"  Reactances1=[ 31 32 33 34 35 36 37 ]  Reactances2=[ 1.305, 0.296, 0.252, 0.474, 0.243, 0.18 ]  dAxisTimeConstants=Short-circuit  qAxisTimeConstants=Open-circuit  TimeConstants1=[]  TimeConstants2=[]  TimeConstants3=[]  TimeConstants4=[]  TimeConstants5=[ 1.01, 0.053, 0.1 ]  TimeConstants6=[]  TimeConstants7=[]  TimeConstants8=[]  StatorResistance=2.8544e-3  Mechanical=[H1 0 2]  PolePairs=2  InitialConditions=[0 -62.5202 1.01055 1.01055 1.01055 8.25986 -111.74 128.26 1.32748]  SetSaturation=off  Saturation=[0.6404,0.7127,0.8441,0.9214,0.9956,1.082,1.19,1.316,1.457;0.7,0.7698,0.8872,0.9466,0.9969,1.046,1.1,1.151,1.201]  LoadFlowParameters=[1 150000000 0 0]  TsPowergui=0  TsBlock=-1  IterativeModel=Trapezoidal non iterative  IterativeDiscreteModel=Trapezoidal non iterative  BusType=PV  Pref=42e6  Qref=0  Qmin=-50000000  Qmax=50000000  PLF=0  QLF=0
      settings: SourceProductBaseCode=PS
  A : PMIOPort  Side=Right
  B : PMIOPort  Port=2  Side=Right
  C : PMIOPort  Port=3  Side=Right
  sm1 : Outport  VectorParamsAs1DForOutWhenUnconnected=off
  wires:
  Synchronous Machine/1 -> Generator Measurements (Output)/1(m)
  Vref (pu)/1 -> ST6C EXCITER-1/1(Vref)
  Governor model with Droop/1(Pmec (pu)) -> Synchronous Machine/1
  wref (pu)/1 -> Governor model with Droop/1(wref (pu)1)
  Ground7/1 -> ST6C EXCITER-1/5(Vstab)
  [QT1st] -> ST6C EXCITER-1/6(QT)
  [It1st] -> ST6C EXCITER-1/3(It)
  [PT1st] -> ST6C EXCITER-1/7(PT)
  ST6C EXCITER-1/1(Efd) -> [Efd1st], Synchronous Machine/2
  Generator Measurements (Output)/2(wm) -> [wm1]
  Generator Measurements (Output)/4(Ifd) -> [Ifd1st]
  Generator Measurements (Output)/5(It) -> [It1st]
  Generator Measurements (Output)/1(sm) -> sm1/1
  Generator Measurements (Output)/7(QT) -> [QT1st]
  Generator Measurements (Output)/6(PT) -> [PT1st]
  Generator Measurements (Output)/3(Vt) -> [Vt1st]
  [wm1] -> Governor model with Droop/2(w (pu))
  [Vt1st] -> ST6C EXCITER-1/2(Vt)
  [Ifd1st] -> ST6C EXCITER-1/4(Ifd)
  [PT1st] -> Governor model with Droop/3(Input)
  connections:
  B/RConn1 -- Synchronous Machine/RConn2
  C/RConn1 -- Synchronous Machine/RConn3
  A/RConn1 -- Synchronous Machine/RConn1
